simulink model "hexMotorModelTestHarness"  (R2024a)
settings: configuration reference "standardSILConfiguraitonParams" (kept outside this file)
undefined symbols (not defined in the file): rpm2radps
settings Model: Creator=jerem  LastModifiedBy=GTAR
settings ConfigSetRef: SourceName=standardSILConfiguraitonParams  SourceLocation=Base Workspace

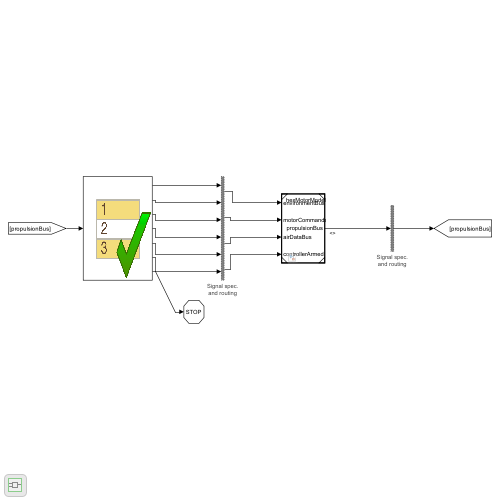
[thumbnail: Simulink's stored preview of the top-level diagram]
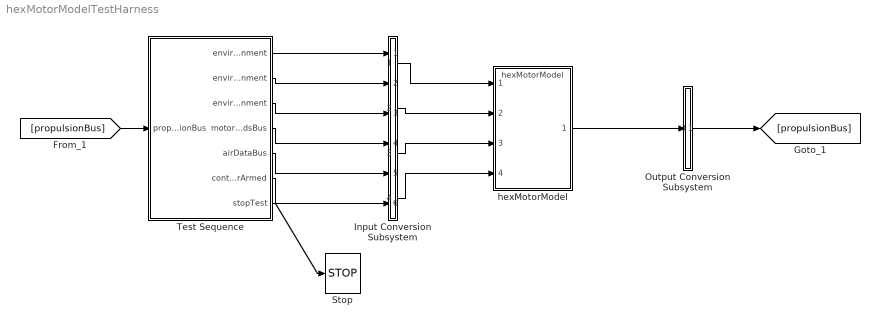
== system hexMotorModelTestHarness ==
  Input Conversion Subsystem : Subsystem  Tag=__SLT_ICS__  Description=|
      | Signal spec.
      | and routing
      settings: AttributesFormatString=%<Description>
  Output Conversion Subsystem : Subsystem  Tag=__SLT_OCS__  Description=|
      | Signal spec.
      | and routing
      mask init:
      | ICDictionary = get_param(bdroot, 'DataDictionary');
      | if isempty(ICDictionary)
      |    ICScope = Simulink.data.BaseWorkspace;
      | else
      |    ICScope = Simulink.data.DataDictionary(ICDictionary);
      | end
      | 
      | IC1 = Simulink.Bus.createMATLABStruct('PropulsionBus', [], [1 1], ICScope);
      settings: AttributesFormatString=%<Description>
  Stop : Stop
  Test Sequence : Test Sequence  TreatAsAtomicUnit=on
  hexMotorModel : ModelReference  ModelNameDialog=hexMotorModel  SimulationMode=Normal  ModelReferenceVersion=1.191
  wires:
  Test Sequence/1(environmentBus_EarthEnvironment) -> Input Conversion Subsystem/1(Inport_1)
  Test Sequence/2(environmentBus_AirEnvironment) -> Input Conversion Subsystem/2(Inport_2)
  Test Sequence/3(environmentBus_TerrainEnvironment) -> Input Conversion Subsystem/3(Inport_3)
  Test Sequence/4(motorCommandsBus) -> Input Conversion Subsystem/4(Inport_4)
  Test Sequence/5(airDataBus) -> Input Conversion Subsystem/5(Inport_5)
  Test Sequence/6(controllerArmed) -> Input Conversion Subsystem/6(Inport_6)
  [propulsionBus] -> Test Sequence/1(propulsionBus)
  Output Conversion Subsystem/1(Outport_1) -> [propulsionBus]
  Input Conversion Subsystem/1(Outport_1) -> hexMotorModel/1
  Input Conversion Subsystem/2(Outport_2) -> hexMotorModel/2
  Input Conversion Subsystem/3(Outport_3) -> hexMotorModel/3
  Input Conversion Subsystem/4(Outport_4) -> hexMotorModel/4
  hexMotorModel/1 -> Output Conversion Subsystem/1(Inport_1)
  Test Sequence/7(stopTest) -> Stop/1

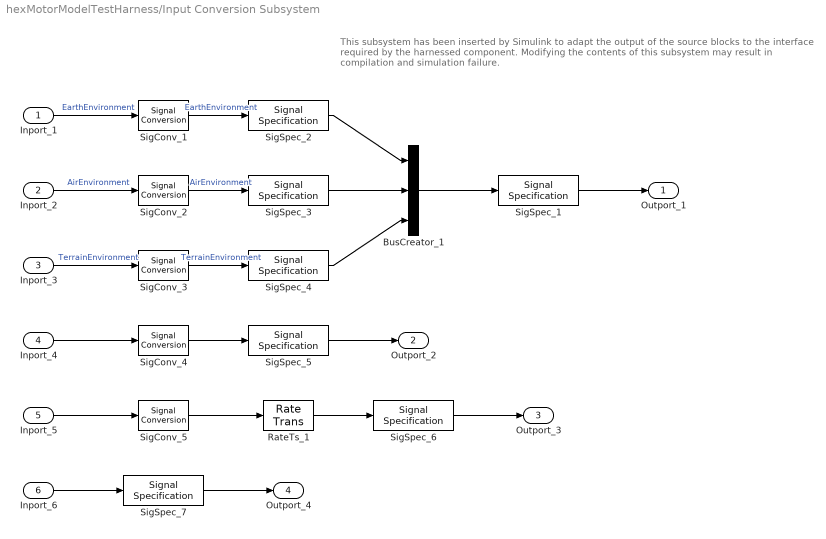
== system hexMotorModelTestHarness/Input Conversion Subsystem ==
  note: This subsystem has been inserted by Simulink to adapt the output of the source blocks to the interface required by the harnessed component.
      |  Modifying the contents of this subsystem may result in compilation and simulation failure.
  Inport_1 : Inport
  Inport_2 : Inport  Port=2
  Inport_3 : Inport  Port=3
  Inport_4 : Inport  Port=4
  Inport_5 : Inport  Port=5
  Inport_6 : Inport  Port=6
  BusCreator_1 : BusCreator  Inputs=3  OutDataTypeStr=Bus: EnvironmentBus
  RateTs_1 : RateTransition  OutPortSampleTime=0.004
  SigConv_1 : SignalConversion  ConversionOutput=Nonvirtual bus  OverrideOpt=off
  SigConv_2 : SignalConversion  ConversionOutput=Nonvirtual bus  OverrideOpt=off
  SigConv_3 : SignalConversion  ConversionOutput=Nonvirtual bus  OverrideOpt=off
  SigConv_4 : SignalConversion  ConversionOutput=Virtual bus  OverrideOpt=off
  SigConv_5 : SignalConversion  ConversionOutput=Virtual bus  OverrideOpt=off
  SigSpec_1 : SignalSpecification  OutDataTypeStr=Bus: EnvironmentBus  SampleTime=[-1, 0]
  SigSpec_2 : SignalSpecification  OutDataTypeStr=Bus: EarthEnvironmentBus  Dimensions=[1]  SampleTime=[-1, 0]  BusOutputAsStruct=on
  SigSpec_3 : SignalSpecification  OutDataTypeStr=Bus: AirEnvironmentBus  Dimensions=[1]  SampleTime=[-1, 0]  BusOutputAsStruct=on
  SigSpec_4 : SignalSpecification  OutDataTypeStr=Bus: TerrainEnvironmentBus  Dimensions=[1]  SampleTime=[-1, 0]  BusOutputAsStruct=on
  SigSpec_5 : SignalSpecification  OutDataTypeStr=Bus: MotorCommandHexBus  SampleTime=[-1, 0]
  SigSpec_6 : SignalSpecification  OutDataTypeStr=Bus: AirDataBus  SampleTime=0.004
  SigSpec_7 : SignalSpecification  OutDataTypeStr=double  Dimensions=[1]  SampleTime=[-1, 0]
  Outport_1 : Outport
  Outport_2 : Outport  Port=2
  Outport_3 : Outport  Port=3
  Outport_4 : Outport  Port=4
  wires:
  SigSpec_1/1 -> Outport_1/1
  BusCreator_1/1 -> SigSpec_1/1
  SigSpec_2/1 -> BusCreator_1/1
  SigConv_1/1 -> SigSpec_2/1  "EarthEnvironment"
  Inport_1/1 -> SigConv_1/1  "EarthEnvironment"
  SigSpec_3/1 -> BusCreator_1/2
  SigConv_2/1 -> SigSpec_3/1  "AirEnvironment"
  Inport_2/1 -> SigConv_2/1  "AirEnvironment"
  SigSpec_4/1 -> BusCreator_1/3
  SigConv_3/1 -> SigSpec_4/1  "TerrainEnvironment"
  Inport_3/1 -> SigConv_3/1  "TerrainEnvironment"
  SigSpec_5/1 -> Outport_2/1
  SigConv_4/1 -> SigSpec_5/1
  Inport_4/1 -> SigConv_4/1
  SigSpec_6/1 -> Outport_3/1
  RateTs_1/1 -> SigSpec_6/1
  SigConv_5/1 -> RateTs_1/1
  Inport_5/1 -> SigConv_5/1
  SigSpec_7/1 -> Outport_4/1
  Inport_6/1 -> SigSpec_7/1

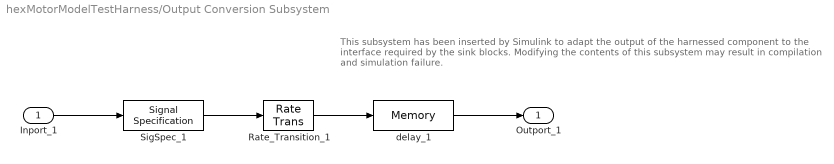
== system hexMotorModelTestHarness/Output Conversion Subsystem ==
  note: This subsystem has been inserted by Simulink to adapt the output of the harnessed component to the interface required by the sink blocks.
      |  Modifying the contents of this subsystem may result in compilation and simulation failure.
  Inport_1 : Inport
  Rate_Transition_1 : RateTransition  OutPortSampleTimeOpt=Inherit
  SigSpec_1 : SignalSpecification  OutDataTypeStr=Bus: PropulsionBus  Dimensions=[1]
  delay_1 : Memory  InitialCondition=IC1
  Outport_1 : Outport
  wires:
  Inport_1/1 -> SigSpec_1/1
  SigSpec_1/1 -> Rate_Transition_1/1
  Rate_Transition_1/1 -> delay_1/1
  delay_1/1 -> Outport_1/1

== stateflow chart hexMotorModelTestHarness/Test Sequence ==
  state Scenario_1
    state Initialize
      %% Initialize data outputs.
      environmentBus_EarthEnvironment.gravityScalar_mps2 = 0;
      environmentBus_EarthEnvironment.worldMagneticFieldInNED_nT = zeros(3,1);
      environmentBus_EarthEnvironment.mulh = zeros(3,1);
      environmentBus_AirEnvironment.airTemperature_K = 0;
      environmentBus_AirEnvironment.airPressure_Pa = 0;
      environmentBus_AirEnvironment.airDensity_kgpm3 = 1.225;
      environmentBus_AirEnvironment.windSpeedInNED_mps = zeros(3,1);
      environmentBus_AirEnvironment.speedOfSound_mps = 0;
      environmentBus_AirEnvironment.windsAloftInNED_mps = zeros(3,1);
      environmentBus_AirEnvironment.gustInNED_mps = zeros(3,1);
      environmentBus_AirEnvironment.turbulenceInNED_mps = zeros(3,1);
      environmentBus_TerrainEnvironment.terrainHeightInNED_m = 0;
      motorCommandsBus.cmdRotor1_nd = 0;
      motorCommandsBus.cmdRotor2_nd = 0;
      motorCommandsBus.cmdRotor3_nd = 0;
      motorCommandsBus.cmdRotor4_nd = 0;
      motorCommandsBus.cmdRotor5_nd = 0;
      motorCommandsBus.cmdRotor6_nd = 0;
      airDataBus.airspeedInBody_mps = zeros(3,1);
      airDataBus.alpha_rad = 0;
      airDataBus.beta_rad = 0;
      controllerArmed = 0;
      stopTest = false;
    state attemptSpinWithoutArm
      motorCommandsBus.cmdRotor1_nd = 1;
      motorCommandsBus.cmdRotor2_nd = 1;
      motorCommandsBus.cmdRotor3_nd = 1;
      motorCommandsBus.cmdRotor4_nd = 1;
      motorCommandsBus.cmdRotor5_nd = 1;
      motorCommandsBus.cmdRotor6_nd = 1;
    state verifyNoSpin
      verify(isClose(sum(propulsionBus.rotorAngVel_radps),0))
      verify(isClose(sum(propulsionBus.engineForcesMoments.forcesInBody_N),0))
      verify(isClose(sum(propulsionBus.engineForcesMoments.momentsInBody_Nm),0))
    state armController
      controllerArmed  = 1;
    state verifyControllerArm
      verify(isClose(sum(propulsionBus.rotorAngVel_radps)/6, 3473 * rpm2radps ))% Check that we have max angular velocity on all rotors (3473 is max RPM)
      verify(propulsionBus.engineForcesMoments.forcesInBody_N(3) < 0)
      verify(isClose(sum(propulsionBus.engineForcesMoments.momentsInBody_Nm(3)), 0))
      maxForce = propulsionBus.engineForcesMoments.forcesInBody_N;
      maxAngVel_radps = propulsionBus.rotorAngVel_radps(1);
    state AttemptOOBCommandOver
      motorCommandsBus.cmdRotor1_nd = 2;
      motorCommandsBus.cmdRotor2_nd = 2;
      motorCommandsBus.cmdRotor3_nd = 2;
      motorCommandsBus.cmdRotor4_nd = 2;
      motorCommandsBus.cmdRotor5_nd = 2;
      motorCommandsBus.cmdRotor6_nd = 2;
    state verifyOutputNoChange
      verify(isClose(propulsionBus.engineForcesMoments.forcesInBody_N(1),maxForce(1)))
      verify(isClose(propulsionBus.engineForcesMoments.forcesInBody_N(2),maxForce(2)))
      verify(isClose(propulsionBus.engineForcesMoments.forcesInBody_N(3),maxForce(3)))
      verify(isClose(maxAngVel_radps,propulsionBus.rotorAngVel_radps(1)))
    state killAllMotorsButCommand1
      motorCommandsBus.cmdRotor2_nd = 0;
      motorCommandsBus.cmdRotor3_nd = 0;
      motorCommandsBus.cmdRotor4_nd = 0;
      motorCommandsBus.cmdRotor5_nd = 0;
      motorCommandsBus.cmdRotor6_nd = 0;
    state verifyMotor1OnlyRunning
      verify(propulsionBus.engineForcesMoments.momentsInBody_Nm(1) < 0) % Motor 1 creates negative rotation about body X-axis
      verify(isClose(propulsionBus.engineForcesMoments.momentsInBody_Nm(2),  0)) %this will change if DFC angle
      verify(propulsionBus.engineForcesMoments.momentsInBody_Nm(3) < 0) % Motor 1 creates negative torque
      verify(isClose(propulsionBus.engineForcesMoments.forcesInBody_N(3),maxForce(3) / 6)) % Verify that the force of only one motor is output
    state testMotor2
      motorCommandsBus.cmdRotor1_nd = 0;
      motorCommandsBus.cmdRotor2_nd = 1;
    state verifyMotor2OnlyRunning
      verify(propulsionBus.engineForcesMoments.momentsInBody_Nm(1) > 0)
      verify(isClose(propulsionBus.engineForcesMoments.momentsInBody_Nm(2),  0)) %this will change if DFC angle
      verify(propulsionBus.engineForcesMoments.momentsInBody_Nm(3) > 0)
      verify(isClose(propulsionBus.engineForcesMoments.forcesInBody_N(3),maxForce(3) / 6)) % Verify that the force of only one motor is output
    state testMotor3
      motorCommandsBus.cmdRotor2_nd = 0;
      motorCommandsBus.cmdRotor3_nd = 1;
    state verifyMotor3
      verify(propulsionBus.engineForcesMoments.momentsInBody_Nm(1) > 0)
      verify(propulsionBus.engineForcesMoments.momentsInBody_Nm(2) > 0)
      verify(propulsionBus.engineForcesMoments.momentsInBody_Nm(3) < 0)
      verify(isClose(propulsionBus.engineForcesMoments.forcesInBody_N(3),maxForce(3) / 6)) % Verify that the force of only one motor is output
    state testMotor4
      motorCommandsBus.cmdRotor3_nd = 0;
      motorCommandsBus.cmdRotor4_nd = 1;
    state verifyMotor4
      verify(propulsionBus.engineForcesMoments.momentsInBody_Nm(1) < 0)
      verify(propulsionBus.engineForcesMoments.momentsInBody_Nm(2) < 0)
      verify(propulsionBus.engineForcesMoments.momentsInBody_Nm(3) > 0)
      verify(isClose(propulsionBus.engineForcesMoments.forcesInBody_N(3),maxForce(3) / 6)) % Verify that the force of only one motor is output
    state testMotor5
      motorCommandsBus.cmdRotor4_nd = 0;
      motorCommandsBus.cmdRotor5_nd = 1;
    state verifyMotor5
      verify(propulsionBus.engineForcesMoments.momentsInBody_Nm(1) < 0)
      verify(propulsionBus.engineForcesMoments.momentsInBody_Nm(2) > 0)
      verify(propulsionBus.engineForcesMoments.momentsInBody_Nm(3) < 0)
      verify(isClose(propulsionBus.engineForcesMoments.forcesInBody_N(3),maxForce(3) / 6)) % Verify that the force of only one motor is output
    state testMotor6
      motorCommandsBus.cmdRotor5_nd = 0;
      motorCommandsBus.cmdRotor6_nd = 1;
    state verifyMotor6
      verify(propulsionBus.engineForcesMoments.momentsInBody_Nm(1) > 0)
      verify(propulsionBus.engineForcesMoments.momentsInBody_Nm(2) < 0)
      verify(propulsionBus.engineForcesMoments.momentsInBody_Nm(3) > 0)
      verify(isClose(propulsionBus.engineForcesMoments.forcesInBody_N(3),maxForce(3) / 6)) % Verify that the force of only one motor is output
    state AttemptOOBCommandUnder
      motorCommandsBus.cmdRotor1_nd = -2;
      motorCommandsBus.cmdRotor2_nd = -2;
      motorCommandsBus.cmdRotor3_nd = -2;
      motorCommandsBus.cmdRotor4_nd = -2;
      motorCommandsBus.cmdRotor5_nd = -2;
      motorCommandsBus.cmdRotor6_nd = -2;
    state verifyOutputZero
      verify(isClose(sum(propulsionBus.rotorAngVel_radps),0))
      verify(isClose(sum(propulsionBus.engineForcesMoments.forcesInBody_N),0))
      verify(isClose(sum(propulsionBus.engineForcesMoments.momentsInBody_Nm),0))
    state EndTest
      stopTest = true;
    (default) -> Initialize
    Initialize -> attemptSpinWithoutArm : [
        | true
        | ]
    attemptSpinWithoutArm -> verifyNoSpin : [
        | after(1,sec)
        | ]
    verifyNoSpin -> armController : [
        | true
        | ]
    armController -> verifyControllerArm : [
        | after(1,sec)
        | ]
    verifyControllerArm -> AttemptOOBCommandOver : [
        | true
        | ]
    AttemptOOBCommandOver -> verifyOutputNoChange : [
        | after(1,sec)
        | ]
    verifyOutputNoChange -> killAllMotorsButCommand1 : [
        | true
        | ]
    killAllMotorsButCommand1 -> verifyMotor1OnlyRunning : [
        | after(1,sec)
        | ]
    verifyMotor1OnlyRunning -> testMotor2 : [
        | true
        | ]
    testMotor2 -> verifyMotor2OnlyRunning : [
        | after(1,sec)
        | ]
    verifyMotor2OnlyRunning -> testMotor3 : [
        | true
        | ]
    testMotor3 -> verifyMotor3 : [
        | after(1,sec)
        | ]
    verifyMotor3 -> testMotor4 : [
        | true
        | ]
    testMotor4 -> verifyMotor4 : [
        | after(1,sec)
        | ]
    verifyMotor4 -> testMotor5 : [
        | true
        | ]
    testMotor5 -> verifyMotor5 : [
        | after(1,sec)
        | ]
    verifyMotor5 -> testMotor6 : [
        | true
        | ]
    testMotor6 -> verifyMotor6 : [
        | after(1,sec)
        | ]
    verifyMotor6 -> AttemptOOBCommandUnder : [
        | true
        | ]
    AttemptOOBCommandUnder -> verifyOutputZero : [
        | after(1, sec)
        | ]
    verifyOutputZero -> EndTest : [
        | true
        | ]
  (default) -> Scenario_1 : {assert(Active_Scenario_Index == 1,'The value of Scenario Parameter ''Active_Scenario_Index'' is not valid. Use the index of the scenario to specify it.')}
  data: propulsionBus input Bus: PropulsionBus size=[1]; environmentBus_EarthEnvironment output Bus: EarthEnvironmentBus size=[1]; environmentBus_AirEnvironment output Bus: AirEnvironmentBus size=[1]; environmentBus_TerrainEnvironment output Bus: TerrainEnvironmentBus size=[1]; motorCommandsBus output Bus: MotorCommandHexBus size=[1]; airDataBus output Bus: AirDataBus size=[1]; controllerArmed output double size=[1]; stopTest output; Active_Scenario_Index parameter =1; rpm2radps parameter; maxAngVel_radps local; maxForce local
